simulink subsystem "ASMController"  (R2023a)
settings: Solver=VariableStepAuto  StartTime=0.0  StopTime=10.0  RelTol=1e-3
undefined symbols (not defined in the file): ASMC
settings Model: Creator=Dell  LastModifiedBy=Dell

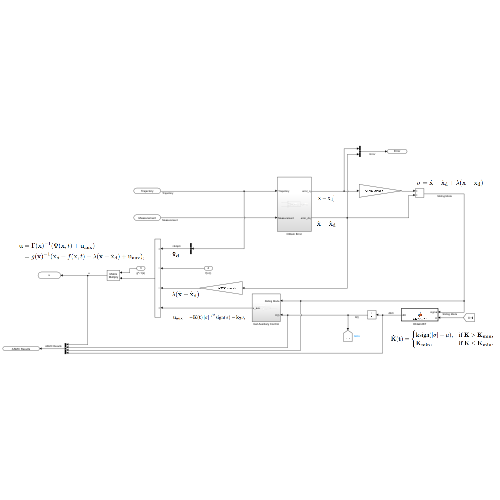
[thumbnail: Simulink's stored preview of the top-level diagram]
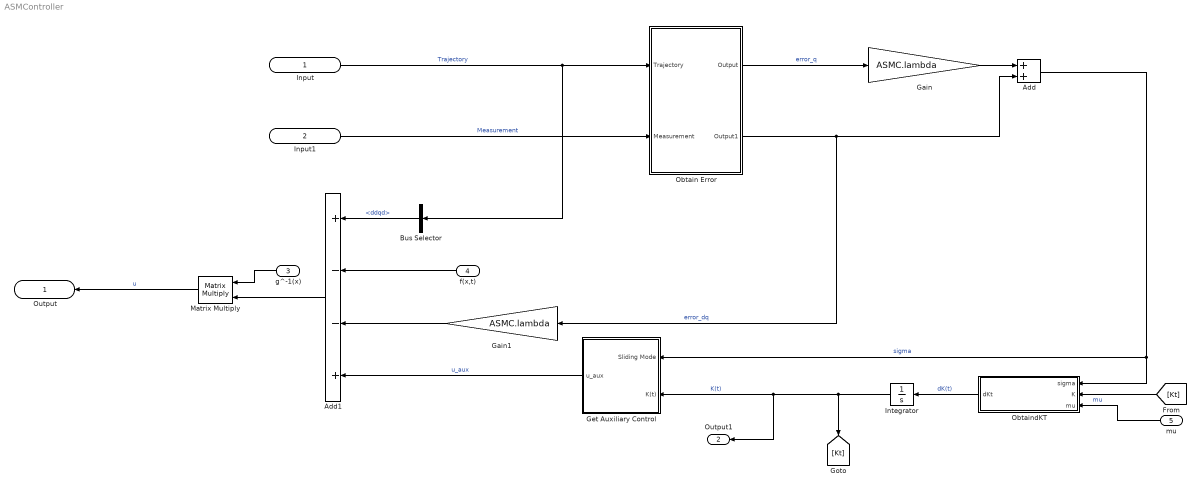
== system ASMController ==
  Input : Inport
  Input1 : Inport  Port=2
  g^-1(x) : Inport  Port=3
  f(x,t) : Inport  Port=4
  mu : Inport  Port=5
  Add : Sum
  Add1 : Sum  Inputs=+--+
  Bus Selector : BusSelector  OutputSignals=ddqd
  Gain : Gain  Gain=ASMC.lambda
  Gain1 : Gain  Gain=ASMC.lambda
  Get Auxiliary Control : Subsystem
  Integrator : Integrator  InitialCondition=ASMC.K0
  Matrix Multiply : Product  Multiplication=Matrix(*)
  Obtain Error : Subsystem
  ObtaindKT : MATLAB Function  TreatAsAtomicUnit=on
  Output : Outport
  Output1 : Outport  Port=2
  wires:
  Input1/1 -> Obtain Error/2(Measurement)  "Measurement"
  Input/1 -> Obtain Error/1(Trajectory), Bus Selector/1  "Trajectory"
  Obtain Error/2(Output1) -> Gain1/1, Add/2  "error_dq"
  Obtain Error/1(Output) -> Gain/1  "error_q"
  Gain/1 -> Add/1
  Add/1 -> ObtaindKT/1(sigma), Get Auxiliary Control/1(Sliding Mode)  "sigma"
  [Kt] -> ObtaindKT/2(K)
  ObtaindKT/1(dKt) -> Integrator/1  "dK(t)"
  Integrator/1 -> [Kt], Get Auxiliary Control/2(K(t)), Output1/1  "K(t)"
  Get Auxiliary Control/1(u_aux) -> Add1/4  "u_aux"
  f(x,t)/1 -> Add1/2
  Gain1/1 -> Add1/3
  g^-1(x)/1 -> Matrix Multiply/1
  Add1/1 -> Matrix Multiply/2
  Matrix Multiply/1 -> Output/1  "u"
  mu/1 -> ObtaindKT/3(mu)  "mu"
  Bus Selector/1 -> Add1/1  "<ddqd>"

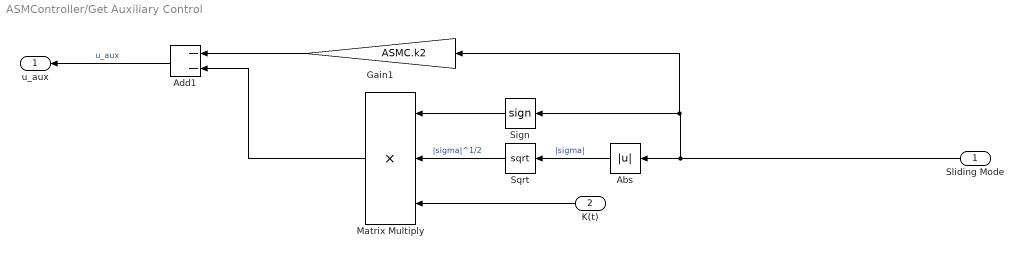
== system ASMController/Get Auxiliary Control ==
  Sliding Mode : Inport
  K(t) : Inport  Port=2
  Abs : Abs  SaturateOnIntegerOverflow=off
  Add1 : Sum  Inputs=--
  Gain1 : Gain  Gain=ASMC.k2
  Matrix Multiply : Product  Inputs=3
  Sign : Signum
  Sqrt : Sqrt
  u_aux : Outport
  wires:
  Add1/1 -> u_aux/1  "u_aux"
  Sqrt/1 -> Matrix Multiply/2  "|sigma|^1/2"
  K(t)/1 -> Matrix Multiply/3
  Sign/1 -> Matrix Multiply/1
  Sliding Mode/1 -> Abs/1, Sign/1, Gain1/1
  Abs/1 -> Sqrt/1  "|sigma|"
  Matrix Multiply/1 -> Add1/2
  Gain1/1 -> Add1/1

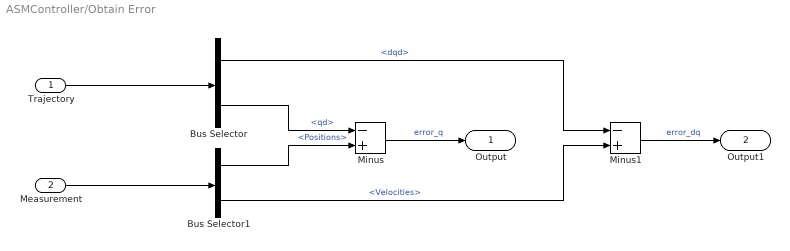
== system ASMController/Obtain Error ==
  Trajectory : Inport
  Measurement : Inport  Port=2
  Bus Selector : BusSelector  OutputSignals=dqd,qd
  Bus Selector1 : BusSelector  OutputSignals=Positions,Velocities
  Minus : Sum  Inputs=-+
  Minus1 : Sum  Inputs=-+
  Output : Outport
  Output1 : Outport  Port=2
  wires:
  Bus Selector1/2 -> Minus1/2  "<Velocities>"
  Bus Selector1/1 -> Minus/2  "<Positions>"
  Minus1/1 -> Output1/1  "error_dq"
  Minus/1 -> Output/1  "error_q"
  Bus Selector/2 -> Minus/1  "<qd>"
  Bus Selector/1 -> Minus1/1  "<dqd>"
  Measurement/1 -> Bus Selector1/1
  Trajectory/1 -> Bus Selector/1

== matlab function ASMController/ObtaindKT ==
  data: sigma input; K input; dKt output; ASMC parameter; mu input
function dKt = ObtainDKt(sigma, K, ASMC, mu)

Kmin = ASMC.Kmin;
k    = ASMC.k;

dKt = zeros(length(K),1);

idx = K > Kmin;

dKt( idx) = k(idx) .* sign( abs(sigma(idx)) - mu(idx) );
dKt(~idx) = Kmin(~idx);

end
